simulink model "P7_Simulink"  (R2023b)
settings: Solver=VariableStepAuto  StartTime=0.0  StopTime=5  RelTol=1e-3
values from neighbouring files (symbols this model uses):
  C1 = 100e-9    (= 1e-07)    [P7_SisElec.m]    (also in P7_parameters.mat)
  C2 = 100e-9    (= 1e-07)    [P7_SisElec.m]    (also in P7_parameters.mat)
  R1 = 5e6    (= 5000000)    [P7_SisElec.m]    (also in P7_parameters.mat)
  R2 = 5e6    (= 5000000)    [P7_SisElec.m]    (also in P7_parameters.mat)
  R3 = 5e6    (= 5000000)    [P7_SisElec.m]    (also in P7_parameters.mat)

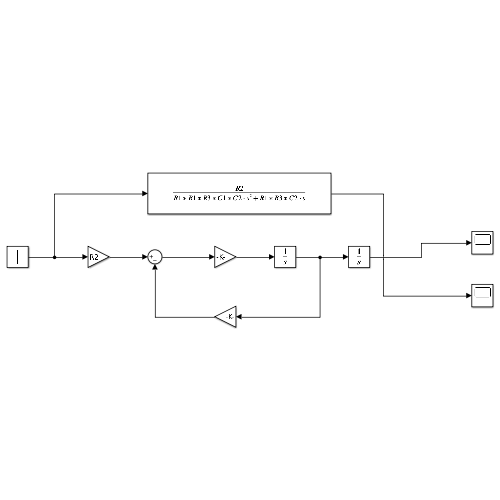
[thumbnail: Simulink's stored preview of the top-level diagram]
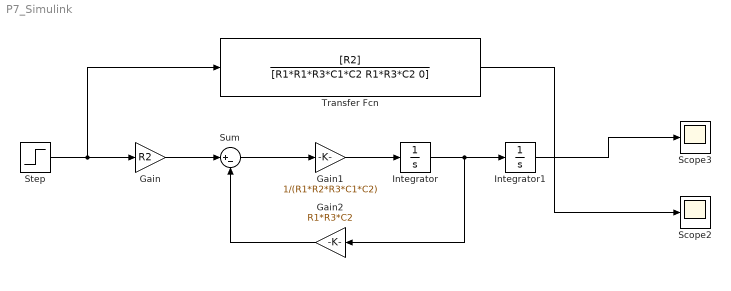
== system P7_Simulink ==
  Gain : Gain  Gain=R2
  Gain1 : Gain  Gain=1/(R1*R2*R3*C1*C2)
  Gain2 : Gain  Gain=R1*R3*C2
  Integrator : Integrator
  Integrator1 : Integrator
  Scope2 : Scope
  Scope3 : Scope
  Step : Step  Time=0  After=5  SampleTime=0
  Sum : Sum  Inputs=|+-
  Transfer Fcn : TransferFcn  Numerator=[R2]  Denominator=[R1*R1*R3*C1*C2 R1*R3*C2 0]
  wires:
  Transfer Fcn/1 -> Scope2/1
  Sum/1 -> Gain1/1
  Integrator/1 -> Integrator1/1, Gain2/1
  Step/1 -> Transfer Fcn/1, Gain/1
  Gain2/1 -> Sum/2
  Gain/1 -> Sum/1
  Integrator1/1 -> Scope3/1
  Gain1/1 -> Integrator/1
